simulink model "CarModel_TestId"  (R2022b)
settings: Solver=VariableStepAuto  StartTime=0.0  StopTime=100  RelTol=1e-3
values from neighbouring files (symbols this model uses):
  DenM = [1; X(1:ModelOrder)]'    [Setup_Id.m]
  InputPower = 1    [Setup_Id.m]
  NumM = X(ModelOrder+1:end)'    [Setup_Id.m]
  Ts = 4    [Setup_Ctrl.m]    (also in Setup_Id.m = 0.5)
libraries: simulink x4
settings Model: Creator=rvilanova  LastModifiedBy=rvilanova

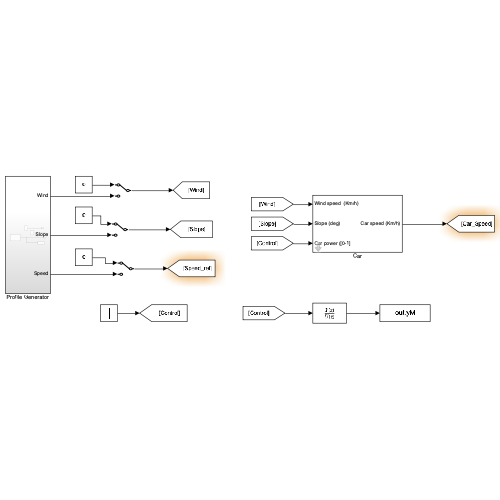
[thumbnail: Simulink's stored preview of the top-level diagram]
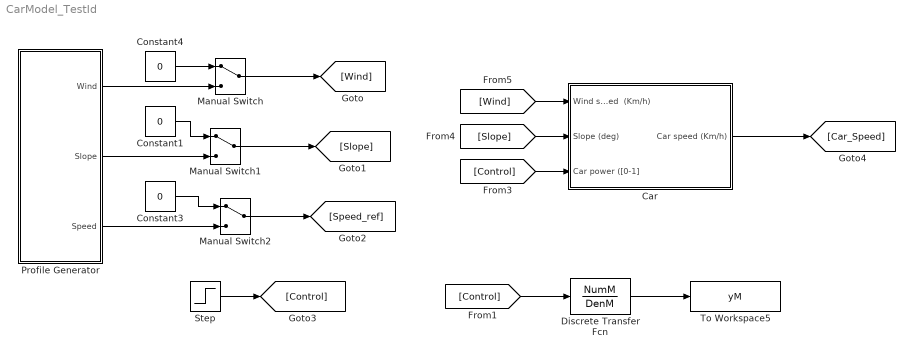
== system CarModel_TestId ==
  Car : Subsystem  mask{M=1000}
      mask prompts: M "Pes del vehicle"
  Constant1 : Constant  Value=0
  Constant3 : Constant  Value=0
  Constant4 : Constant  Value=0
  Discrete Transfer Fcn : DiscreteTransferFcn  Numerator=NumM  Denominator=DenM  SampleTime=Ts
  Manual Switch : ManualSwitch
  Manual Switch1 : ManualSwitch
  Manual Switch2 : ManualSwitch
  Profile Generator : Subsystem
  Step : Step  Time=10  After=InputPower  SampleTime=0
  To Workspace5 : ToWorkspace  VariableName=yM  SaveFormat=Timeseries  SampleTime=Ts
  wires:
  Step/1 -> [Control]
  Manual Switch1/1 -> [Slope]
  Manual Switch2/1 -> [Speed_ref]
  Profile Generator/3(Speed) -> Manual Switch2/2
  Profile Generator/1(Wind) -> Manual Switch/2
  Manual Switch/1 -> [Wind]
  Constant4/1 -> Manual Switch/1
  Profile Generator/2(Slope) -> Manual Switch1/2
  Constant3/1 -> Manual Switch2/1
  Constant1/1 -> Manual Switch1/1
  [Control] -> Car/3(Car power ([0-1])
  [Slope] -> Car/2(Slope (deg))
  Car/1(Car speed (Km/h)) -> [Car_Speed]
  [Wind] -> Car/1(Wind speed  (Km/h))
  [Control] -> Discrete Transfer Fcn/1
  Discrete Transfer Fcn/1 -> To Workspace5/1

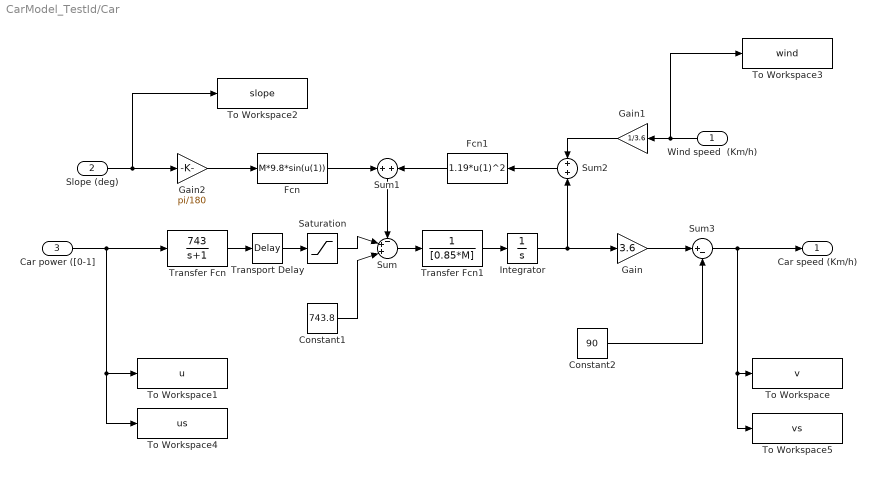
== system CarModel_TestId/Car ==
  Wind speed  (Km/h) : Inport
  Slope (deg) : Inport  Port=2
  Car power ([0-1] : Inport  Port=3
  Constant1 : Constant  Value=743.8
  Constant2 : Constant  Value=90
  Fcn : Fcn  Expr=M*9.8*sin(u(1))
  Fcn1 : Fcn  Expr=1.19*u(1)^2
  Gain : Gain  Gain=3.6
  Gain1 : Gain  Gain=1/3.6
  Gain2 : Gain  Gain=pi/180
  Integrator : Integrator  InitialCondition=25
  Saturation : Saturate  UpperLimit=3000  LowerLimit=-3000
  Sum : Sum  Inputs=-++|  InputSameDT=on  SaturateOnIntegerOverflow=on  OutDataTypeStr=Inherit: Same as first input
  Sum1 : Sum  InputSameDT=on  SaturateOnIntegerOverflow=on  OutDataTypeStr=Inherit: Same as first input
  Sum2 : Sum  Inputs=+|+  InputSameDT=on  SaturateOnIntegerOverflow=on  OutDataTypeStr=Inherit: Same as first input
  Sum3 : Sum  Inputs=|+-  InputSameDT=on  SaturateOnIntegerOverflow=on  OutDataTypeStr=Inherit: Same as first input
  To Workspace : ToWorkspace  VariableName=v  SaveFormat=Timeseries  SampleTime=-1
  To Workspace1 : ToWorkspace  VariableName=u  SaveFormat=Timeseries  SampleTime=-1
  To Workspace2 : ToWorkspace  VariableName=slope  SaveFormat=Timeseries  SampleTime=-1
  To Workspace3 : ToWorkspace  VariableName=wind  SaveFormat=Timeseries  SampleTime=-1
  To Workspace4 : ToWorkspace  VariableName=us  SaveFormat=Timeseries  SampleTime=Ts
  To Workspace5 : ToWorkspace  VariableName=vs  SaveFormat=Timeseries  SampleTime=Ts
  Transfer Fcn : TransferFcn  Numerator=[743]  Denominator=[1 1]
  Transfer Fcn1 : TransferFcn  Denominator=[0.85*M]
  Transport Delay : TransportDelay  DelayTime=0.3
  Car speed (Km/h) : Outport
  wires:
  Slope (deg)/1 -> To Workspace2/1, Gain2/1
  Gain2/1 -> Fcn/1
  Gain1/1 -> Sum2/1
  Wind speed  (Km/h)/1 -> To Workspace3/1, Gain1/1
  Transfer Fcn/1 -> Transport Delay/1
  Transport Delay/1 -> Saturation/1
  Sum/1 -> Transfer Fcn1/1
  Transfer Fcn1/1 -> Integrator/1
  Fcn1/1 -> Sum1/2
  Sum2/1 -> Fcn1/1
  Sum1/1 -> Sum/1
  Fcn/1 -> Sum1/1
  Integrator/1 -> Gain/1, Sum2/2
  Car power ([0-1]/1 -> To Workspace4/1, To Workspace1/1, Transfer Fcn/1
  Saturation/1 -> Sum/2
  Constant1/1 -> Sum/3
  Gain/1 -> Sum3/1
  Sum3/1 -> To Workspace5/1, To Workspace/1, Car speed (Km/h)/1
  Constant2/1 -> Sum3/2

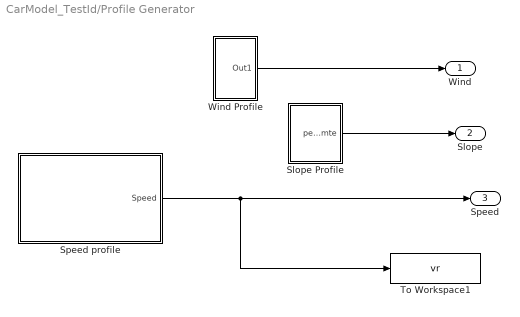
== system CarModel_TestId/Profile Generator ==
  Slope Profile : Subsystem
  Speed profile : Subsystem
  To Workspace1 : ToWorkspace  VariableName=vr  SaveFormat=Timeseries  SampleTime=-1
  Wind Profile : Subsystem
  Wind : Outport
  Slope : Outport  Port=2
  Speed : Outport  Port=3
  wires:
  Slope Profile/1(pendiemte) -> Slope/1
  Wind Profile/1(Out1) -> Wind/1
  Speed profile/1(Speed) -> Speed/1, To Workspace1/1

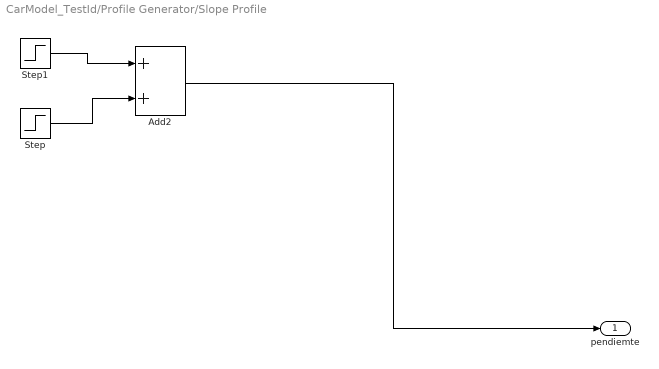
== system CarModel_TestId/Profile Generator/Slope Profile ==
  Add2 : Sum
  Step : Step  Time=400  After=5*(pi/180)  SampleTime=0
  Step1 : Step  Time=350  After=-5*(pi/180)  SampleTime=0
  pendiemte : Outport
  wires:
  Step1/1 -> Add2/1
  Step/1 -> Add2/2
  Add2/1 -> pendiemte/1

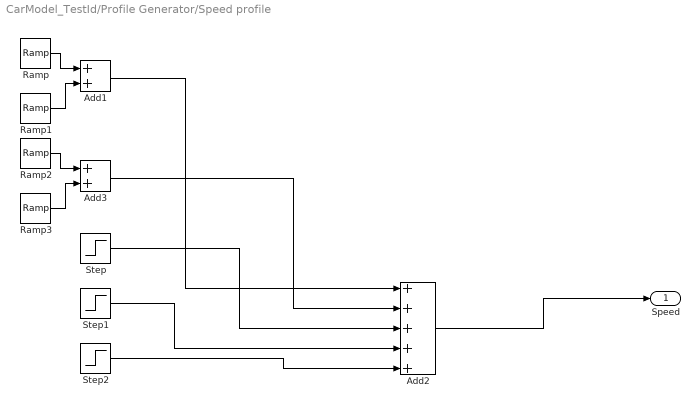
== system CarModel_TestId/Profile Generator/Speed profile ==
  Add1 : Sum
  Add2 : Sum  Inputs=+++++
  Add3 : Sum
  Ramp : simulink/Sources/Ramp  slope=0.5  start=20  InitialOutput=0
  Ramp1 : simulink/Sources/Ramp  slope=-0.5  start=60  InitialOutput=0
  Ramp2 : simulink/Sources/Ramp  slope=-0.5  start=260  InitialOutput=0
  Ramp3 : simulink/Sources/Ramp  slope=0.5  start=300  InitialOutput=0
  Step : Step  Time=500  After=-10  SampleTime=0
  Step1 : Step  Time=600  After=20  SampleTime=0
  Step2 : Step  Time=700  After=-10  SampleTime=0
  Speed : Outport
  wires:
  Ramp3/1 -> Add3/2
  Add3/1 -> Add2/2
  Step2/1 -> Add2/5
  Step1/1 -> Add2/4
  Add2/1 -> Speed/1
  Ramp2/1 -> Add3/1
  Ramp/1 -> Add1/1
  Ramp1/1 -> Add1/2
  Add1/1 -> Add2/1
  Step/1 -> Add2/3

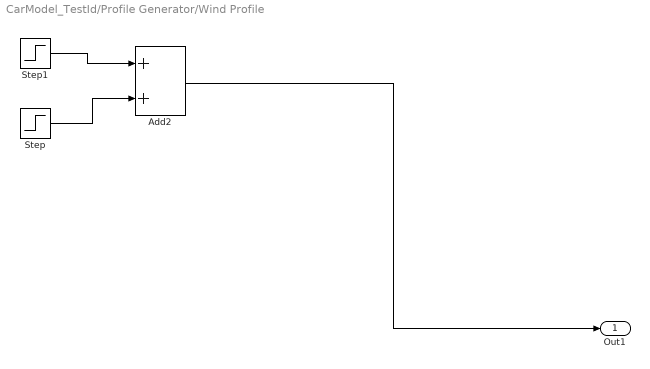
== system CarModel_TestId/Profile Generator/Wind Profile ==
  Add2 : Sum
  Step : Step  Time=150  After=-20  SampleTime=0
  Step1 : Step  Time=100  After=20  SampleTime=0
  Out1 : Outport
  wires:
  Step1/1 -> Add2/1
  Step/1 -> Add2/2
  Add2/1 -> Out1/1
